simulink model "controller_test"  (Simulink 7.9)
settings: Solver=ode4  StartTime=0.0  StopTime=10  FixedStep=0.01  RelTol=1e-3
undefined symbols (not defined in the file or in its folder): DiscIntNeverNeededParam, fundamental_sample_time, trajectory_time
libraries: simulink x3
settings Model: Creator=Bazs  LastModifiedBy=Bazs
settings OptimizationCC: BlockReduction=off
settings DebuggingCC: MultiTaskRateTransMsg=warning

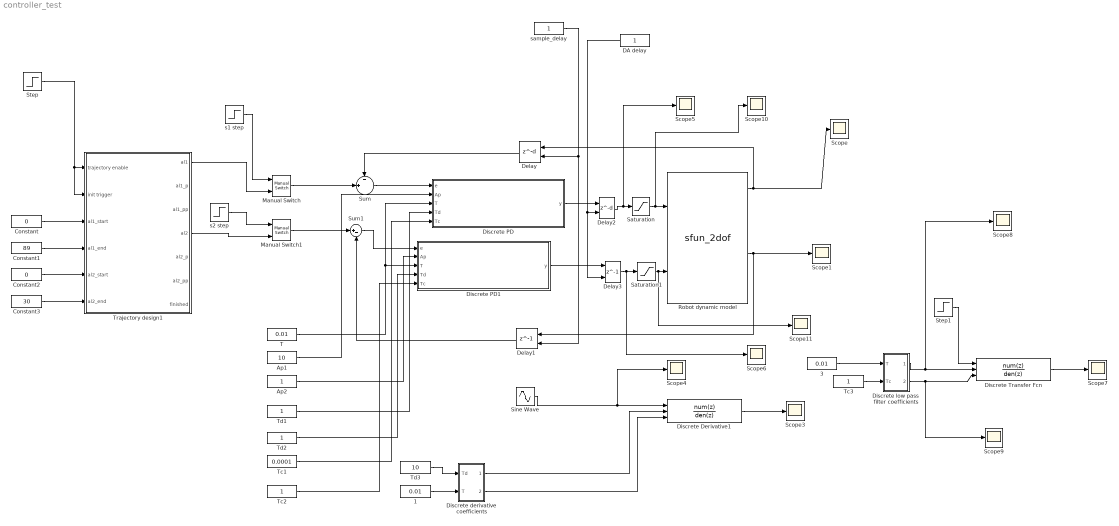
== system controller_test ==
  1 : Constant  Value=0.01
  3 : Constant  Value=0.01  SampleTime=0.01
  Ap1 : Constant  Value=10
  Ap2 : Constant
  Constant : Constant  Value=0
  Constant1 : Constant  Value=89
  Constant2 : Constant  Value=0
  Constant3 : Constant  Value=30
  DA delay : Constant
  Delay : Delay  DelayLengthSource=Input port  DelayLength=1
      settings: InputPortMap=u0,p1
  Delay1 : Delay  DelayLength=1  InitialConditionSource=Input port
      settings: InputPortMap=u0,p4
  Delay2 : Delay  DelayLengthSource=Input port  DelayLength=1
      settings: InputPortMap=u0,p1
  Delay3 : Delay  DelayLength=1  InitialConditionSource=Input port
      settings: InputPortMap=u0,p4
  Discrete Derivative1 : DiscreteTransferFcn  NumeratorSource=Input port  DenominatorSource=Input port  SampleTime=fundamental_sample_time  a0EqualsOne=on
      settings: InputPortMap=u0,p1,p3
  Discrete Transfer Fcn : DiscreteTransferFcn  NumeratorSource=Input port  Numerator=[0.01 0]  DenominatorSource=Input port  Denominator=[1.01 -1]  SampleTime=0.01  a0EqualsOne=on
      settings: InputPortMap=u0,p1,p3
  Discrete PD : Subsystem
  Discrete PD1 : Subsystem
  Discrete derivative coefficients : Subsystem
  Discrete low pass filter coefficients : Subsystem
  Manual Switch : simulink/Signal Routing/Manual Switch  sw=0  action=0  varsize=off
  Manual Switch1 : simulink/Signal Routing/Manual Switch  sw=0  action=0  varsize=off
  Robot dynamic model : M-S-Function  FunctionName=sfun_2dof  Parameters=0.4, 1, 0.2, 0.5, 0.033, 0.004166
  Saturation : Saturate  UpperLimit=1.751  LowerLimit=-1.751
  Saturation1 : Saturate  UpperLimit=1.751  LowerLimit=-1.751
  Scope{,1,3..11} (11 alike) : Scope
      Scope settings: YMin=14  YMax=23.5
      Scope1 settings: TimeRange=50  YMin=-40  YMax=100
      Scope10 settings: YMin=9e-05  YMax=0.00022  SaveName=ScopeData13
      Scope11 settings: TimeRange=10  YMin=-150  YMax=100  SaveName=ScopeData14
      Scope3 settings: TimeRange=50  YMin=-10  YMax=10  SaveName=ScopeData3
      Scope4 settings: TimeRange=50  YMin=-1  YMax=1  SaveName=ScopeData4
      Scope5 settings: YMin=9e-05  YMax=0.00022  SaveName=ScopeData6
      Scope6 settings: TimeRange=10  YMin=-150  YMax=100  SaveName=ScopeData7
      Scope7 settings: TimeRange=10  YMin=0.88  YMax=1  SaveName=ScopeData8
      Scope8 settings: TimeRange=10  YMin=0.979  YMax=1  SaveName=ScopeData9
      Scope9 settings: TimeRange=10  YMin=-1  YMax=1.1  SaveName=ScopeData10
  Sine Wave : Sin  SampleTime=0
  Step : Step  Time=0.01  SampleTime=0
  Step1 : Step  Time=0.01  SampleTime=0
  Sum : Sum  Inputs=-|+||
  Sum1 : Sum  Inputs=|+-
  T : Constant  Value=0.01
  Tc1 : Constant  Value=0.0001
  Tc2 : Constant
  Tc3 : Constant  SampleTime=0.01
  Td1 : Constant
  Td2 : Constant
  Td3 : Constant  Value=10
  Trajectory design1 : Subsystem
  s1 step : Step  Time=0.01  After=20  SampleTime=0
  s2 step : Step  Time=0.01  After=30  SampleTime=0
  sample_delay : Constant
  wires:
  Discrete PD/1(y) -> Delay2/1
  Step/1 -> Trajectory design1/1(trajectory enable), Trajectory design1/2(init trigger)
  Constant/1 -> Trajectory design1/3(al1_start)
  Constant1/1 -> Trajectory design1/4(al1_end)
  Constant2/1 -> Trajectory design1/5(al2_start)
  Constant3/1 -> Trajectory design1/6(al2_end)
  Robot dynamic model/1 -> Delay/1, Scope/1
  Robot dynamic model/3 -> Scope1/1, Delay1/1
  Sum/1 -> Discrete PD/1(e)
  Sum1/1 -> Discrete PD1/1(e)
  Ap1/1 -> Discrete PD/2(Ap)
  Ap2/1 -> Discrete PD1/2(Ap)
  T/1 -> Discrete PD/3(T), Discrete PD1/3(T)
  Td1/1 -> Discrete PD/4(Td)
  Td2/1 -> Discrete PD1/4(Td)
  Tc1/1 -> Discrete PD/5(Tc)
  Tc2/1 -> Discrete PD1/5(Tc)
  Discrete derivative coefficients/1(Num) -> Discrete Derivative1/2
  Discrete derivative coefficients/2(Den) -> Discrete Derivative1/3
  Td3/1 -> Discrete derivative coefficients/1(Td)
  1/1 -> Discrete derivative coefficients/2(T)
  Discrete Derivative1/1 -> Scope3/1
  Delay/1 -> Sum/1
  Delay1/1 -> Sum1/2
  Delay2/1 -> Scope5/1, Saturation/1
  Discrete PD1/1(y) -> Delay3/1
  Delay3/1 -> Scope6/1, Saturation1/1
  sample_delay/1 -> Delay/2, Delay1/2
  DA delay/1 -> Delay2/2, Delay3/2
  Tc3/1 -> Discrete low pass filter coefficients/2(Tc)
  3/1 -> Discrete low pass filter coefficients/1(T)
  Step1/1 -> Discrete Transfer Fcn/1
  Discrete low pass filter coefficients/1(Num) -> Scope8/1, Discrete Transfer Fcn/2
  Discrete low pass filter coefficients/2(Den) -> Scope9/1, Discrete Transfer Fcn/3
  Sine Wave/1 -> Discrete Derivative1/1, Scope4/1
  Discrete Transfer Fcn/1 -> Scope7/1
  s1 step/1 -> Manual Switch/1
  Manual Switch/1 -> Sum/2
  Trajectory design1/1(al1) -> Manual Switch/2
  Manual Switch1/1 -> Sum1/1
  Trajectory design1/4(al2) -> Manual Switch1/2
  s2 step/1 -> Manual Switch1/1
  Saturation/1 -> Robot dynamic model/1, Scope10/1
  Saturation1/1 -> Robot dynamic model/2, Scope11/1

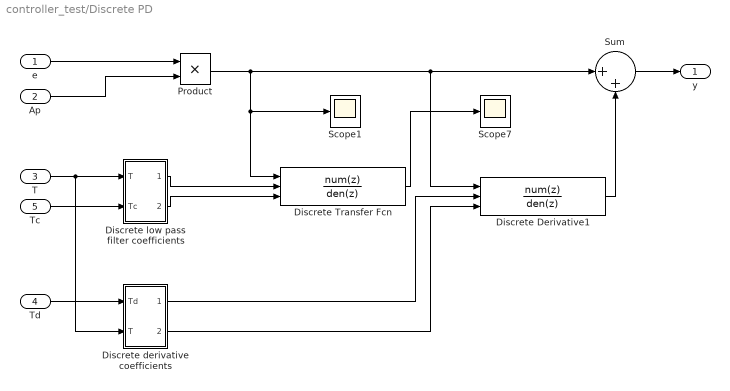
== system controller_test/Discrete PD ==
  e : Inport
  Ap : Inport  Port=2
  T : Inport  Port=3
  Td : Inport  Port=4
  Tc : Inport  Port=5
  Discrete Derivative1 : DiscreteTransferFcn  NumeratorSource=Input port  DenominatorSource=Input port  SampleTime=fundamental_sample_time  a0EqualsOne=on
      settings: InputPortMap=u0,p1,p3
  Discrete Transfer Fcn : DiscreteTransferFcn  NumeratorSource=Input port  DenominatorSource=Input port  SampleTime=fundamental_sample_time  a0EqualsOne=on
      settings: InputPortMap=u0,p1,p3
  Discrete derivative coefficients : Subsystem
  Discrete low pass filter coefficients : Subsystem
  Product : Product  RndMeth=Zero
  Scope1 : Scope
      settings: TimeRange=10  YMin=-0.15  YMax=0.7  SaveName=ScopeData12
  Scope7 : Scope
      settings: TimeRange=10  YMin=-0.15  YMax=0.7  SaveName=ScopeData11
  Sum : Sum  Inputs=|++
  y : Outport
  wires:
  Product/1 -> Discrete Transfer Fcn/1, Scope1/1, Sum/1, Discrete Derivative1/1
  Discrete low pass filter coefficients/1(Num) -> Discrete Transfer Fcn/2
  Discrete low pass filter coefficients/2(Den) -> Discrete Transfer Fcn/3
  e/1 -> Product/1
  Sum/1 -> y/1
  Ap/1 -> Product/2
  T/1 -> Discrete derivative coefficients/2(T), Discrete low pass filter coefficients/1(T)
  Tc/1 -> Discrete low pass filter coefficients/2(Tc)
  Td/1 -> Discrete derivative coefficients/1(Td)
  Discrete Derivative1/1 -> Sum/2
  Discrete derivative coefficients/1(Num) -> Discrete Derivative1/2
  Discrete derivative coefficients/2(Den) -> Discrete Derivative1/3
  Discrete Transfer Fcn/1 -> Scope7/1

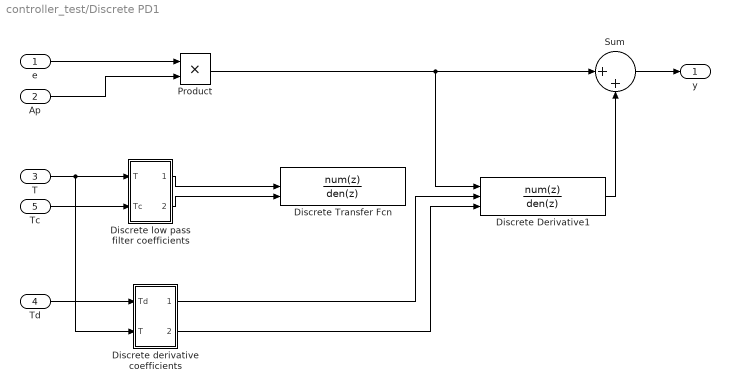
== system controller_test/Discrete PD1 ==
  e : Inport
  Ap : Inport  Port=2
  T : Inport  Port=3
  Td : Inport  Port=4
  Tc : Inport  Port=5
  Discrete Derivative1 : DiscreteTransferFcn  NumeratorSource=Input port  DenominatorSource=Input port  SampleTime=fundamental_sample_time  a0EqualsOne=on
      settings: InputPortMap=u0,p1,p3
  Discrete Transfer Fcn : DiscreteTransferFcn  NumeratorSource=Input port  DenominatorSource=Input port  SampleTime=0.01  a0EqualsOne=on
      settings: InputPortMap=u0,p1,p3
  Discrete derivative coefficients : Subsystem
  Discrete low pass filter coefficients : Subsystem
  Product : Product  RndMeth=Zero
  Sum : Sum  Inputs=|++
  y : Outport
  wires:
  Discrete derivative coefficients/2(Den) -> Discrete Derivative1/3
  Discrete derivative coefficients/1(Num) -> Discrete Derivative1/2
  Discrete Derivative1/1 -> Sum/2
  Td/1 -> Discrete derivative coefficients/1(Td)
  Tc/1 -> Discrete low pass filter coefficients/2(Tc)
  T/1 -> Discrete derivative coefficients/2(T), Discrete low pass filter coefficients/1(T)
  Ap/1 -> Product/2
  Sum/1 -> y/1
  e/1 -> Product/1
  Discrete low pass filter coefficients/2(Den) -> Discrete Transfer Fcn/3
  Discrete low pass filter coefficients/1(Num) -> Discrete Transfer Fcn/2
  Product/1 -> Sum/1, Discrete Derivative1/1

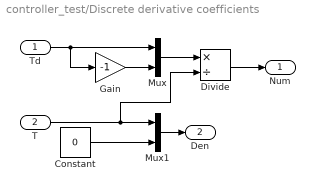
== system controller_test/Discrete derivative coefficients ==
  Td : Inport
  T : Inport  Port=2
  Constant : Constant  Value=0
  Divide : Product  Inputs=*/
  Gain : Gain  Gain=-1
  Mux : Mux  Inputs=2
  Mux1 : Mux  Inputs=2
  Num : Outport
  Den : Outport  Port=2
  wires:
  Td/1 -> Mux/1, Gain/1
  Gain/1 -> Mux/2
  Constant/1 -> Mux1/2
  Mux1/1 -> Den/1
  T/1 -> Mux1/1, Divide/2
  Mux/1 -> Divide/1
  Divide/1 -> Num/1

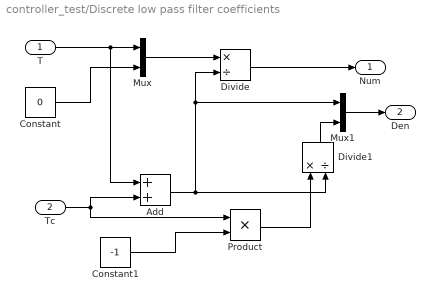
== system controller_test/Discrete low pass filter coefficients ==
  T : Inport
  Tc : Inport  Port=2
  Add : Sum
  Constant : Constant  Value=0
  Constant1 : Constant  Value=-1
  Divide : Product  Inputs=*/
  Divide1 : Product  Inputs=*/
  Mux : Mux  Inputs=2
  Mux1 : Mux  Inputs=2
  Product : Product  RndMeth=Zero
  Num : Outport
  Den : Outport  Port=2
  wires:
  T/1 -> Mux/1, Add/1
  Constant/1 -> Mux/2
  Tc/1 -> Product/1, Add/2
  Mux1/1 -> Den/1
  Constant1/1 -> Product/2
  Add/1 -> Mux1/1, Divide/2, Divide1/2
  Mux/1 -> Divide/1
  Divide/1 -> Num/1
  Product/1 -> Divide1/1
  Divide1/1 -> Mux1/2

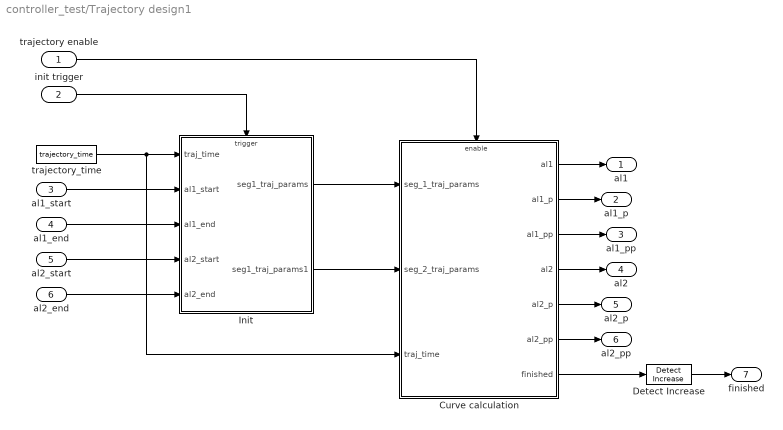
== system controller_test/Trajectory design1 ==
  trajectory enable : Inport
  init trigger : Inport  Port=2
  al1_start : Inport  Port=3
  al1_end : Inport  Port=4
  al2_start : Inport  Port=5
  al2_end : Inport  Port=6
  Curve calculation : Subsystem
  Detect Increase : simulink/Logic and Bit Operations/Detect Increase  vinit=0.0  InputProcessing=Inherited  OutDataTypeStr=uint8
  Init : Subsystem
  trajectory_time : Constant  Value=trajectory_time
  al1 : Outport
  al1_p : Outport  Port=2
  al1_pp : Outport  Port=3
  al2 : Outport  Port=4
  al2_p : Outport  Port=5
  al2_pp : Outport  Port=6
  finished : Outport  Port=7
  wires:
  trajectory_time/1 -> Curve calculation/3(traj_time), Init/1(traj_time)
  al1_end/1 -> Init/3(al1_end)
  Init/2(seg1_traj_params1) -> Curve calculation/2(seg_2_traj_params)
  Init/1(seg1_traj_params) -> Curve calculation/1(seg_1_traj_params)
  trajectory enable/1 -> Curve calculation/Enable
  Curve calculation/1(al1) -> al1/1
  Curve calculation/2(al1_p) -> al1_p/1
  al1_start/1 -> Init/2(al1_start)
  Curve calculation/3(al1_pp) -> al1_pp/1
  Curve calculation/4(al2) -> al2/1
  Curve calculation/5(al2_p) -> al2_p/1
  Curve calculation/6(al2_pp) -> al2_pp/1
  al2_start/1 -> Init/4(al2_start)
  al2_end/1 -> Init/5(al2_end)
  init trigger/1 -> Init/Trigger
  Curve calculation/7(finished) -> Detect Increase/1
  Detect Increase/1 -> finished/1

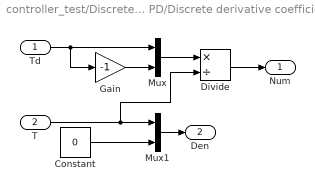
== system controller_test/Discrete PD/Discrete derivative coefficients ==
  Td : Inport
  T : Inport  Port=2
  Constant : Constant  Value=0
  Divide : Product  Inputs=*/
  Gain : Gain  Gain=-1
  Mux : Mux  Inputs=2
  Mux1 : Mux  Inputs=2
  Num : Outport
  Den : Outport  Port=2
  wires:
  Td/1 -> Mux/1, Gain/1
  Gain/1 -> Mux/2
  Constant/1 -> Mux1/2
  Mux1/1 -> Den/1
  T/1 -> Mux1/1, Divide/2
  Mux/1 -> Divide/1
  Divide/1 -> Num/1

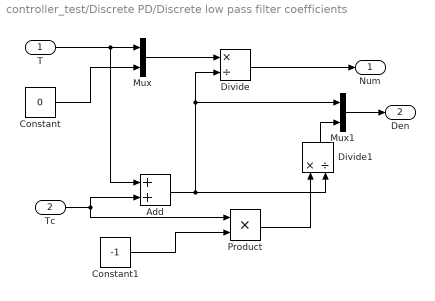
== system controller_test/Discrete PD/Discrete low pass filter coefficients ==
  T : Inport
  Tc : Inport  Port=2
  Add : Sum
  Constant : Constant  Value=0
  Constant1 : Constant  Value=-1
  Divide : Product  Inputs=*/
  Divide1 : Product  Inputs=*/
  Mux : Mux  Inputs=2
  Mux1 : Mux  Inputs=2
  Product : Product  RndMeth=Zero
  Num : Outport
  Den : Outport  Port=2
  wires:
  T/1 -> Mux/1, Add/1
  Constant/1 -> Mux/2
  Tc/1 -> Product/1, Add/2
  Mux1/1 -> Den/1
  Constant1/1 -> Product/2
  Add/1 -> Mux1/1, Divide/2, Divide1/2
  Mux/1 -> Divide/1
  Divide/1 -> Num/1
  Product/1 -> Divide1/1
  Divide1/1 -> Mux1/2

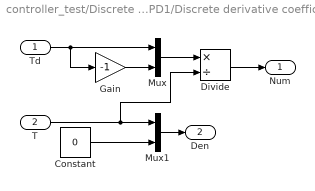
== system controller_test/Discrete PD1/Discrete derivative coefficients ==
  Td : Inport
  T : Inport  Port=2
  Constant : Constant  Value=0
  Divide : Product  Inputs=*/
  Gain : Gain  Gain=-1
  Mux : Mux  Inputs=2
  Mux1 : Mux  Inputs=2
  Num : Outport
  Den : Outport  Port=2
  wires:
  Td/1 -> Mux/1, Gain/1
  Gain/1 -> Mux/2
  Constant/1 -> Mux1/2
  Mux1/1 -> Den/1
  T/1 -> Mux1/1, Divide/2
  Mux/1 -> Divide/1
  Divide/1 -> Num/1

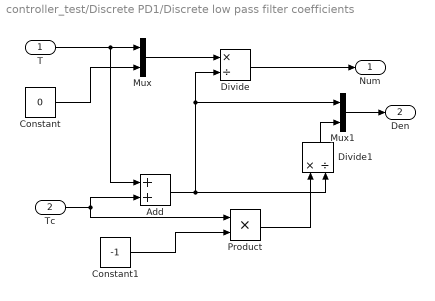
== system controller_test/Discrete PD1/Discrete low pass filter coefficients ==
  T : Inport
  Tc : Inport  Port=2
  Add : Sum
  Constant : Constant  Value=0
  Constant1 : Constant  Value=-1
  Divide : Product  Inputs=*/
  Divide1 : Product  Inputs=*/
  Mux : Mux  Inputs=2
  Mux1 : Mux  Inputs=2
  Product : Product  RndMeth=Zero
  Num : Outport
  Den : Outport  Port=2
  wires:
  T/1 -> Mux/1, Add/1
  Constant/1 -> Mux/2
  Tc/1 -> Product/1, Add/2
  Mux1/1 -> Den/1
  Constant1/1 -> Product/2
  Add/1 -> Mux1/1, Divide/2, Divide1/2
  Mux/1 -> Divide/1
  Divide/1 -> Num/1
  Product/1 -> Divide1/1
  Divide1/1 -> Mux1/2

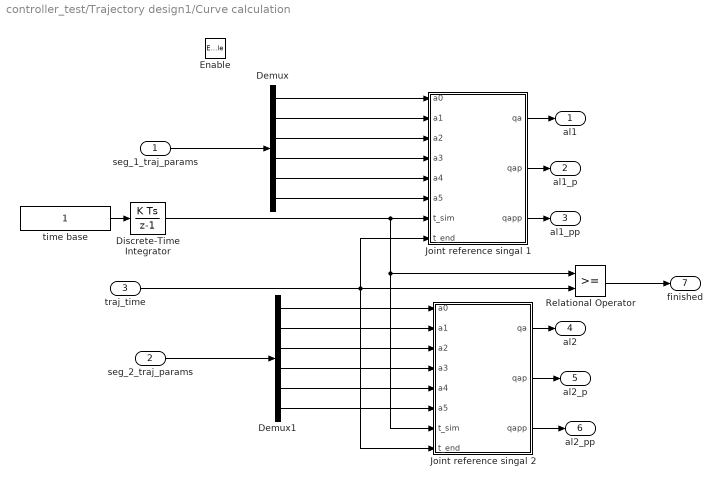
== system controller_test/Trajectory design1/Curve calculation ==
  seg_1_traj_params : Inport
  seg_2_traj_params : Inport  Port=2
  traj_time : Inport  Port=3
  Enable : EnablePort  StatesWhenEnabling=reset
  Demux : Demux  Outputs=6
  Demux1 : Demux  Outputs=6
  Discrete-Time Integrator : DiscreteIntegrator  SampleTime=-1  ICPrevOutput=DiscIntNeverNeededParam  ICPrevScaledInput=DiscIntNeverNeededParam
  Joint reference singal 1 : MATLAB Function  TreatAsAtomicUnit=on
  Joint reference singal 2 : MATLAB Function  TreatAsAtomicUnit=on
  Relational Operator : RelationalOperator  OutDataTypeStr=boolean
  time base : Constant
  al1 : Outport
  al1_p : Outport  Port=2
  al1_pp : Outport  Port=3
  al2 : Outport  Port=4
  al2_p : Outport  Port=5
  al2_pp : Outport  Port=6
  finished : Outport  Port=7
  wires:
  Joint reference singal 1/1(qa) -> al1/1
  Joint reference singal 1/2(qap) -> al1_p/1
  Joint reference singal 1/3(qapp) -> al1_pp/1
  Joint reference singal 2/1(qa) -> al2/1
  Discrete-Time Integrator/1 -> Joint reference singal 1/7(t_sim), Joint reference singal 2/7(t_sim), Relational Operator/1
  time base/1 -> Discrete-Time Integrator/1
  Demux/1 -> Joint reference singal 1/1(a0)
  Demux/2 -> Joint reference singal 1/2(a1)
  Demux/3 -> Joint reference singal 1/3(a2)
  Demux/4 -> Joint reference singal 1/4(a3)
  Demux/5 -> Joint reference singal 1/5(a4)
  Demux/6 -> Joint reference singal 1/6(a5)
  Demux1/1 -> Joint reference singal 2/1(a0)
  Demux1/2 -> Joint reference singal 2/2(a1)
  Demux1/3 -> Joint reference singal 2/3(a2)
  Demux1/4 -> Joint reference singal 2/4(a3)
  Demux1/5 -> Joint reference singal 2/5(a4)
  Demux1/6 -> Joint reference singal 2/6(a5)
  seg_1_traj_params/1 -> Demux/1
  seg_2_traj_params/1 -> Demux1/1
  traj_time/1 -> Joint reference singal 1/8(t_end), Joint reference singal 2/8(t_end), Relational Operator/2
  Relational Operator/1 -> finished/1
  Joint reference singal 2/2(qap) -> al2_p/1
  Joint reference singal 2/3(qapp) -> al2_pp/1

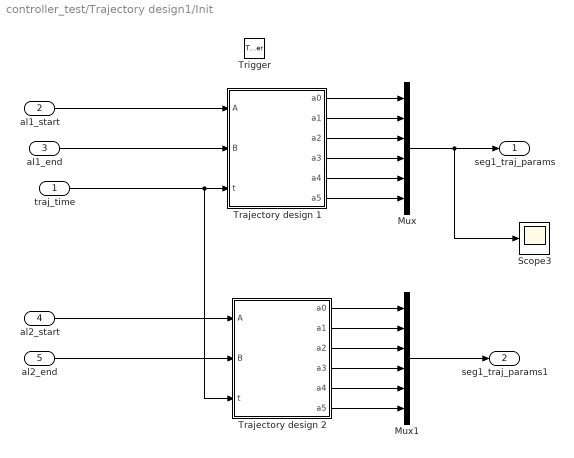
== system controller_test/Trajectory design1/Init ==
  traj_time : Inport
  al1_start : Inport  Port=2  LatchByDelayingOutsideSignal=on
  al1_end : Inport  Port=3
  al2_start : Inport  Port=4  LatchByDelayingOutsideSignal=on
  al2_end : Inport  Port=5
  Trigger : TriggerPort
  Mux : Mux  Inputs=6
  Mux1 : Mux  Inputs=6
  Scope3 : Scope
      settings: YMin=38  YMax=42  SaveName=ScopeData5
  Trajectory design 1 : MATLAB Function  TreatAsAtomicUnit=on
  Trajectory design 2 : MATLAB Function  TreatAsAtomicUnit=on
  seg1_traj_params : Outport
  seg1_traj_params1 : Outport  Port=2
  wires:
  al1_start/1 -> Trajectory design 1/1(A)
  al1_end/1 -> Trajectory design 1/2(B)
  al2_start/1 -> Trajectory design 2/1(A)
  al2_end/1 -> Trajectory design 2/2(B)
  traj_time/1 -> Trajectory design 1/3(t), Trajectory design 2/3(t)
  Trajectory design 1/1(a0) -> Mux/1
  Trajectory design 1/2(a1) -> Mux/2
  Trajectory design 1/3(a2) -> Mux/3
  Trajectory design 1/4(a3) -> Mux/4
  Trajectory design 1/5(a4) -> Mux/5
  Trajectory design 1/6(a5) -> Mux/6
  Trajectory design 2/1(a0) -> Mux1/1
  Trajectory design 2/2(a1) -> Mux1/2
  Trajectory design 2/3(a2) -> Mux1/3
  Trajectory design 2/4(a3) -> Mux1/4
  Trajectory design 2/5(a4) -> Mux1/5
  Trajectory design 2/6(a5) -> Mux1/6
  Mux/1 -> seg1_traj_params/1, Scope3/1
  Mux1/1 -> seg1_traj_params1/1

== matlab function Trajectory design1/Curve calculation/Joint reference singal 1 ==
  settings: fimath=|
      | fimath(...
      | 'RoundMode', 'floor',...
      | 'OverflowMode', 'wrap',...
      | 'ProductMode', 'KeepLSB', 'ProductWordLength', 32,...
      | 'SumMode', 'KeepLSB', 'SumWordLength', 32,...
      | 'CastBeforeSum', false)
  data: a0 input double; a1 input double; a2 input double; a3 input double; a4 input double; a5 input double; t_sim input double; qa output double; qap output double; qapp output double; t_end input double
function [qa,qap,qapp] = fcn(a0,a1,a2,a3,a4,a5,t_sim,t_end)
% This block supports an embeddable subset of the MATLAB language.
% See the help menu for details. 
if (t_sim>=t_end) 
    t_sim = t_end;
end   
T = [t_sim^5/20 t_sim^4/12 t_sim^3/6 t_sim^2/2 t_sim 1;...
    t_sim^4/4 t_sim^3/3 t_sim^2/2 t_sim 1 0;...
    t_sim^3 t_sim^2 t_sim 1 0 0];
Q = T*[a0;a1;a2;a3;a4;a5];

qa = Q(1);
qap = Q(2);
qapp = Q(3);

== matlab function Trajectory design1/Curve calculation/Joint reference singal 2 ==
  settings: fimath=|
      | fimath(...
      | 'RoundMode', 'floor',...
      | 'OverflowMode', 'wrap',...
      | 'ProductMode', 'KeepLSB', 'ProductWordLength', 32,...
      | 'SumMode', 'KeepLSB', 'SumWordLength', 32,...
      | 'CastBeforeSum', false)
  data: a0 input double; a1 input double; a2 input double; a3 input double; a4 input double; a5 input double; t_sim input double; qa output double; qap output double; qapp output double; t_end input double
function [qa,qap,qapp] = fcn(a0,a1,a2,a3,a4,a5,t_sim,t_end)
% This block supports an embeddable subset of the MATLAB language.
% See the help menu for details. 
if (t_sim>=t_end) 
    t_sim = t_end;
end   
T = [t_sim^5/20 t_sim^4/12 t_sim^3/6 t_sim^2/2 t_sim 1;...
    t_sim^4/4 t_sim^3/3 t_sim^2/2 t_sim 1 0;...
    t_sim^3 t_sim^2 t_sim 1 0 0];
Q = T*[a0;a1;a2;a3;a4;a5];

qa = Q(1);
qap = Q(2);
qapp = Q(3);

== matlab function Trajectory design1/Init/Trajectory design 1 ==
  settings: fimath=|
      | fimath(...
      | 'RoundMode', 'floor',...
      | 'OverflowMode', 'wrap',...
      | 'ProductMode', 'KeepLSB', 'ProductWordLength', 32,...
      | 'SumMode', 'KeepLSB', 'SumWordLength', 32,...
      | 'CastBeforeSum', false)
  data: A input double; B input double; t input double; a0 output double; a1 output double; a2 output double; a3 output double; a4 output double; a5 output double
function [a0,a1,a2,a3,a4,a5] = fcn(A,B,t)
% This block supports an embeddable subset of the MATLAB language.
% See the help menu for details. 
T = [t^5/20 t^4/12 t^3/6 t^2/2 t 1;t^4/4 t^3/3 t^2/2 t 1 0;t^3 t^2 t 1 0 0;0 0 0 0 0 1;0 0 0 0 1 0;0 0 0 1 0 0];
Ao = inv(T)*[B;0;0;A;0;0];
a0=Ao(1);
a1=Ao(2);
a2=Ao(3);
a3=Ao(4);
a4=Ao(5);
a5=Ao(6);

== matlab function Trajectory design1/Init/Trajectory design 2 ==
  settings: fimath=|
      | fimath(...
      | 'RoundMode', 'floor',...
      | 'OverflowMode', 'wrap',...
      | 'ProductMode', 'KeepLSB', 'ProductWordLength', 32,...
      | 'SumMode', 'KeepLSB', 'SumWordLength', 32,...
      | 'CastBeforeSum', false)
  data: A input double; B input double; t input double; a0 output double; a1 output double; a2 output double; a3 output double; a4 output double; a5 output double
function [a0,a1,a2,a3,a4,a5] = fcn(A,B,t)
% This block supports an embeddable subset of the MATLAB language.
% See the help menu for details. 
T = [t^5/20 t^4/12 t^3/6 t^2/2 t 1;t^4/4 t^3/3 t^2/2 t 1 0;t^3 t^2 t 1 0 0;0 0 0 0 0 1;0 0 0 0 1 0;0 0 0 1 0 0];
Ao = inv(T)*[B;0;0;A;0;0];
a0=Ao(1);
a1=Ao(2);
a2=Ao(3);
a3=Ao(4);
a4=Ao(5);
a5=Ao(6);
